simulink model "sampleModel2038"  (R2023a)
settings: Solver=VariableStepAuto  StartTime=0.0  StopTime=10.0  RelTol=1e-3
libraries: hdlsllib x8, simulink x2
settings Model: Creator=user1  LastModifiedBy=user1

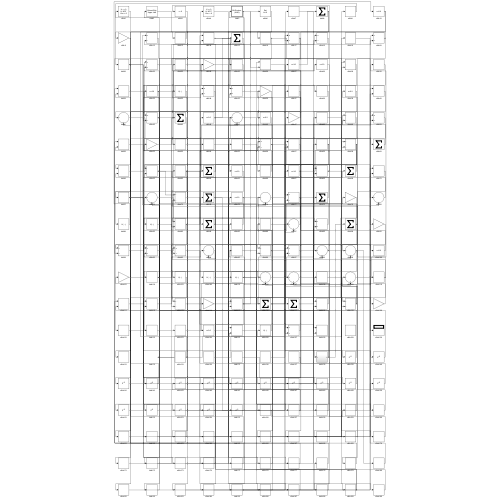
[thumbnail: Simulink's stored preview of the top-level diagram]
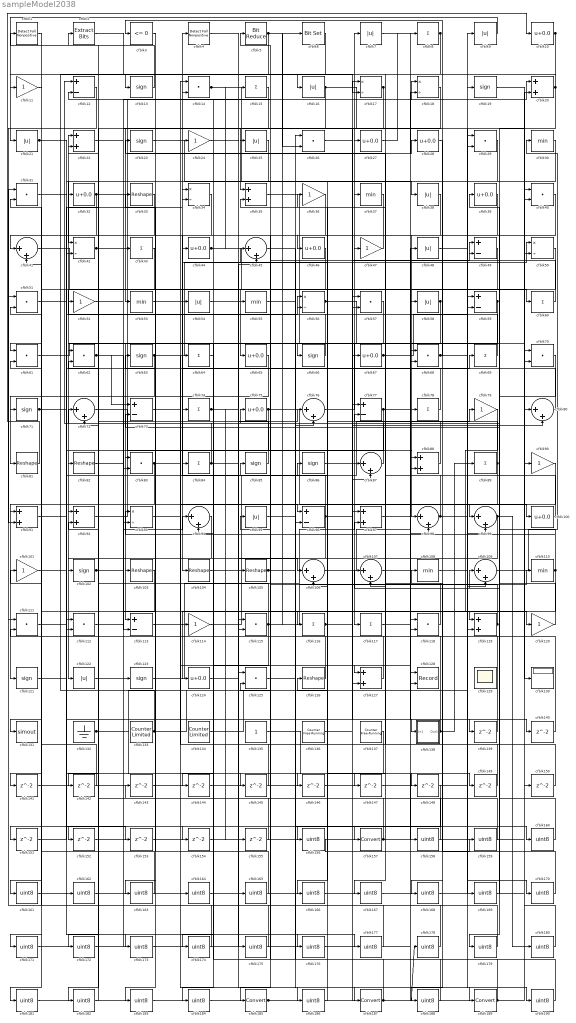
== system sampleModel2038 ==
  cfblk1 : hdlsllib/Logic and Bit Operations/Detect Fall Nonpositive  vinit=0  OutDataTypeStr=boolean
  cfblk{10,27..28,32,39,44,46,65,67,75,100,124} (12 alike) : Bias  Bias=0.0  SaturateOnIntegerOverflow=off
  cfblk{11,24,36,47,52,79,90,101,114,120} (10 alike) : Gain
  cfblk{13,19,23,63,66,71,85..86,102,121,123} (11 alike) : Signum
  cfblk{33,81..82,103..105,126} (7 alike) : Reshape
  cfblk{41,45,72,76,80,87,94,98..99,106..107,109} (12 alike) : Sum  Inputs=|++
  cfblk{30,37,53,55,108,110} (6 alike) : MinMax
  cfblk{14,26,29,31,40,51,57,61..62,68,70,83,111..112,115,118,125} (17 alike) : DotProduct  OutDataTypeStr=Inherit: Inherit via internal rule
  cfblk{12,49,59,73,77,96,113} (7 alike) : Sum  Inputs=+-
  cfblk{8,15,43,60,64,69,74,78,84,89,116..117} (12 alike) : Sum  Inputs=+
  cfblk{20,22,35,88,91..92,97,119,127} (9 alike) : Sum
  cfblk{7,9,16,21,25,38,48,54,58,95,122} (11 alike) : Abs  SaturateOnIntegerOverflow=off
  cfblk128 : Record  FileSettingsInternal="{\"entries\":[{\"content\":{\"excelSettings\":{\"content\":{},\"type\":\"Streamout.ExcelSettings\"}},\"type\":\"Streamout.FileSettingStorage\",\"uuid\":\"\"}],\"packageUris\":[\"http:\\/\\/schema.mathworks.com\\/mf0\\/streamout_blocks\\/R2020a\"],\"version\":\"1.0\"}"  Layout=[1 1]  SignalsInternal="{\"entries\":[{\"content\":{\"signals\":[{\"content\":{\"blockPath\":[],\"dimensions\":[1],\"domain\":\"\",\"lineColor\":\"#a2142f\",\"plots\":[1],\"port\":1,\"signalID\":6186,\"signalName\":\"XY Graph:1\"},\"type\":\"RecordBlkView.Signal\",\"uuid\":\"\"},{\"content\":{\"blockPath\":[],\"dimensions\":[1],\"domain\":\"\",\"lineColor\":\"#139fff\",\"plots\":[1],\"port\":2,\"signalID\":6189,\"signalName\":\"XY Graph:2\"},\"type\":\"RecordBlkView.Signal\",\"uuid\":\"\"}]},\"type\":\"RecordBlkView.InputSignals\",\"uuid\":\"\"}],\"packageUris\":[\"http:\\/\\/schema.mathworks.com\\/mf0\\/streamout_blocks\\/R2020a\"],\"version\":\"1.0\"}"  VisualizationBindings="{\"xyplotplugin\":{\"info\":[{\"series\":[{\"bindingParametersList\":[{\"parameter\":\"X-Axis\",\"signalID\":6186,\"signalName\":\"XY Graph:1\"},{\"parameter\":\"Y-Axis\",\"signalID\":6189,\"signalName\":\"XY Graph:2\"}],\"seriesID\":36534}],\"subplotID\":1}]}}"  CompatibilityTag=XY  st=-1
  cfblk129 : Scope
      settings: Floating=on
  cfblk130 : Display
  cfblk131 : ToWorkspace  VariableName=simout  SaveFormat=Timeseries  SampleTime=-1
  cfblk132 : Ground
  cfblk133 : hdlsllib/Sources/Counter Limited  uplimit=7  tsamp=-1
  cfblk134 : hdlsllib/Sources/Counter Limited  uplimit=7  tsamp=-1
  cfblk135 : Constant  SampleTime=-1
  cfblk136 : hdlsllib/Sources/Counter Free-Running  NumBits=16  tsamp=-1
  cfblk137 : hdlsllib/Sources/Counter Free-Running  NumBits=16  tsamp=-1
  cfblk138 : Subsystem
      settings: LibrarySourceBlock=|
      | hdlsllib/Ports &
      | Subsystems/Subsystem
  cfblk{139..155} (17 alike) : Delay  SampleTime=1
  cfblk{156,158..184,186,188,190} (31 alike) : DataTypeConversion  OutDataTypeStr=uint8  SaturateOnIntegerOverflow=off  RndMeth=Floor
  cfblk{157,185,187,189} (4 alike) : DataTypeConversion  SaturateOnIntegerOverflow=off  RndMeth=Floor
  cfblk{17..18,34,42,50,56,93} (7 alike) : Product  Inputs=*/  RndMeth=Zero  SaturateOnIntegerOverflow=on
  cfblk2 : simulink/Logic and Bit Operations/Extract Bits  bitsToExtract=Upper half  numBits=8  bitIdxRange=[0 7]  outScalingMode=Preserve fixed-point scaling
      settings: LibrarySourceBlock=|
      | hdlsllib/Logic and Bit
      | Operations/Extract Bits
  cfblk3 : hdlsllib/Logic and Bit Operations/Compare To Zero  relop=<=  OutDataTypeStr=boolean
  cfblk4 : hdlsllib/Logic and Bit Operations/Detect Fall Nonpositive  vinit=0  OutDataTypeStr=boolean
  cfblk5 : hdlsllib/Logic and Bit Operations/Bit Reduce  mode=AND
  cfblk6 : simulink/Logic and Bit Operations/Bit Set  iBit=0
      settings: LibrarySourceBlock=|
      | hdlsllib/Logic and Bit
      | Operations/Bit Set
  wires:
  cfblk27/1 -> cfblk8/1
  cfblk78/1 -> cfblk7/1
  cfblk85/1 -> cfblk22/1
  cfblk114/1 -> cfblk79/1
  cfblk98/1 -> cfblk27/1, cfblk109/2
  cfblk84/1 -> cfblk12/1, cfblk119/2
  cfblk133/1 -> cfblk13/1, cfblk45/2
  cfblk20/1 -> cfblk99/1, cfblk11/1
  cfblk68/1 -> cfblk3/1, cfblk170/1
  cfblk79/1 -> cfblk120/1
  cfblk89/1 -> cfblk121/1, cfblk44/1
  cfblk75/1 -> cfblk100/1, cfblk112/2
  cfblk96/1 -> cfblk4/1, cfblk128/2, cfblk144/1
  cfblk49/1 -> cfblk122/1
  cfblk9/1 -> cfblk21/1
  cfblk63/1 -> cfblk50/1, cfblk83/1, cfblk127/1, cfblk83/2
  cfblk87/1 -> cfblk75/1
  cfblk109/1 -> cfblk30/1
  cfblk92/1 -> cfblk28/1
  cfblk53/1 -> cfblk104/1
  cfblk18/1 -> cfblk82/1
  cfblk81/1 -> cfblk10/1
  cfblk80/1 -> cfblk34/1
  cfblk76/1 -> cfblk47/1
  cfblk15/1 -> cfblk35/1
  cfblk37/1 -> cfblk84/1
  cfblk69/1 -> cfblk22/2
  cfblk5/1 -> cfblk26/2, cfblk183/1
  cfblk50/1 -> cfblk65/1
  cfblk61/1 -> cfblk66/1
  cfblk42/1 -> cfblk18/1, cfblk142/1
  cfblk59/1 -> cfblk117/1, cfblk167/1, cfblk168/1
  cfblk35/1 -> cfblk130/1
  cfblk40/1 -> cfblk98/1
  cfblk58/1 -> cfblk113/1, cfblk114/1
  cfblk115/1 -> cfblk110/1, cfblk6/1, cfblk72/1, cfblk184/1
  cfblk13/1 -> cfblk1/1
  cfblk65/1 -> cfblk81/1
  cfblk23/1 -> cfblk77/1
  cfblk119/1 -> cfblk5/1, cfblk107/1
  cfblk21/1 -> cfblk145/1, cfblk146/1
  cfblk17/1 -> cfblk53/1, cfblk127/2
  cfblk19/1 -> cfblk80/1
  cfblk10/1 -> cfblk91/1, cfblk115/2
  cfblk3/1 -> cfblk103/1
  cfblk47/1 -> cfblk41/1
  cfblk46/1 -> cfblk102/1
  cfblk88/1 -> cfblk37/1
  cfblk134/1 -> cfblk59/1
  cfblk102/1 -> cfblk94/1, cfblk62/2
  cfblk120/1 -> cfblk74/1
  cfblk14/1 -> cfblk38/1, cfblk50/2
  cfblk99/1 -> cfblk152/1, cfblk180/1
  cfblk118/1 -> cfblk23/1
  cfblk1/1 -> cfblk131/1
  cfblk22/1 -> cfblk25/1
  cfblk138/1(Out1) -> cfblk63/1, cfblk72/2, cfblk89/1
  cfblk116/1 -> cfblk49/1, cfblk80/2
  cfblk7/1 -> cfblk128/1
  cfblk32/1 -> cfblk18/2, cfblk61/1
  cfblk83/1 -> cfblk56/1, cfblk93/2
  cfblk104/1 -> cfblk76/1
  cfblk60/1 -> cfblk12/2
  cfblk34/1 -> cfblk92/1
  cfblk67/1 -> cfblk19/1, cfblk107/2
  cfblk132/1 -> cfblk97/1, cfblk175/1
  cfblk100/1 -> cfblk35/2
  cfblk30/1 -> cfblk42/1
  cfblk112/1 -> cfblk20/1
  cfblk77/1 -> cfblk48/1, cfblk94/2
  cfblk71/1 -> cfblk138/1(In1), cfblk34/2, cfblk153/1
  cfblk127/1 -> cfblk92/2
  cfblk123/1 -> cfblk97/2
  cfblk136/1 -> cfblk67/1
  cfblk122/1 -> cfblk123/1
  cfblk73/1 -> cfblk96/1
  cfblk91/1 -> cfblk69/1
  cfblk64/1 -> cfblk14/2
  cfblk62/1 -> cfblk119/1, cfblk73/1
  cfblk11/1 -> cfblk71/1
  cfblk16/1 -> cfblk59/2, cfblk62/1
  cfblk24/1 -> cfblk187/1
  cfblk107/1 -> cfblk68/1
  cfblk126/1 -> cfblk32/1
  cfblk44/1 -> cfblk90/1, cfblk15/1
  cfblk12/1 -> cfblk91/2
  cfblk26/1 -> cfblk60/1
  cfblk74/1 -> cfblk106/1, cfblk155/1
  cfblk41/1 -> cfblk87/2
  cfblk95/1 -> cfblk189/1
  cfblk105/1 -> cfblk148/1, cfblk149/1
  cfblk38/1 -> cfblk46/1
  cfblk51/1 -> cfblk56/2
  cfblk36/1 -> cfblk185/1
  cfblk8/1 -> cfblk16/1, cfblk147/1
  cfblk82/1 -> cfblk113/2
  cfblk72/1 -> cfblk88/1
  cfblk106/1 -> cfblk49/2
  cfblk56/1 -> cfblk116/1, cfblk118/1
  cfblk113/1 -> cfblk124/1
  cfblk52/1 -> cfblk54/1
  cfblk54/1 -> cfblk96/2
  cfblk125/1 -> cfblk157/1
  cfblk110/1 -> cfblk73/2, cfblk93/1, cfblk174/1
  cfblk66/1 -> cfblk45/1
  cfblk121/1 -> cfblk85/1
  cfblk2/1 -> cfblk17/2
  cfblk25/1 -> cfblk42/2
  cfblk117/1 -> cfblk88/2
  cfblk45/1 -> cfblk68/2
  cfblk97/1 -> cfblk139/1
  cfblk139/1 -> cfblk41/2
  cfblk86/1 -> cfblk140/1
  cfblk140/1 -> cfblk51/2
  cfblk39/1 -> cfblk141/1
  cfblk141/1 -> cfblk76/2
  cfblk142/1 -> cfblk61/2
  cfblk144/1 -> cfblk118/2
  cfblk145/1 -> cfblk14/1
  cfblk146/1 -> cfblk98/2
  cfblk147/1 -> cfblk99/2
  cfblk149/1 -> cfblk77/2
  cfblk150/1 -> cfblk115/1
  cfblk6/1 -> cfblk151/1
  cfblk151/1 -> cfblk112/1
  cfblk152/1 -> cfblk20/2
  cfblk153/1 -> cfblk87/1
  cfblk90/1 -> cfblk154/1
  cfblk154/1 -> cfblk17/1
  cfblk155/1 -> cfblk33/1
  cfblk137/1 -> cfblk156/1
  cfblk157/1 -> cfblk2/1, cfblk106/2
  cfblk135/1 -> cfblk158/1
  cfblk158/1 -> cfblk125/1
  cfblk156/1 -> cfblk159/1
  cfblk159/1 -> cfblk125/2
  cfblk55/1 -> cfblk160/1
  cfblk160/1 -> cfblk39/1
  cfblk103/1 -> cfblk161/1
  cfblk161/1 -> cfblk55/1
  cfblk101/1 -> cfblk162/1
  cfblk162/1 -> cfblk40/2
  cfblk94/1 -> cfblk163/1
  cfblk163/1 -> cfblk101/1
  cfblk143/1 -> cfblk164/1
  cfblk164/1 -> cfblk40/1
  cfblk4/1 -> cfblk165/1
  cfblk165/1 -> cfblk143/1
  cfblk29/1 -> cfblk166/1
  cfblk166/1 -> cfblk9/1
  cfblk167/1 -> cfblk29/1
  cfblk168/1 -> cfblk29/2
  cfblk108/1 -> cfblk169/1
  cfblk169/1 -> cfblk109/1
  cfblk170/1 -> cfblk108/1
  cfblk43/1 -> cfblk171/1
  cfblk171/1 -> cfblk58/1
  cfblk33/1 -> cfblk172/1
  cfblk172/1 -> cfblk43/1
  cfblk111/1 -> cfblk173/1
  cfblk173/1 -> cfblk105/1
  cfblk174/1 -> cfblk111/1
  cfblk175/1 -> cfblk111/2
  cfblk31/1 -> cfblk176/1
  cfblk176/1 -> cfblk86/1
  cfblk124/1 -> cfblk177/1
  cfblk177/1 -> cfblk31/1
  cfblk178/1 -> cfblk31/2
  cfblk70/1 -> cfblk179/1
  cfblk179/1 -> cfblk51/1
  cfblk180/1 -> cfblk70/1
  cfblk148/1 -> cfblk181/1
  cfblk181/1 -> cfblk70/2
  cfblk57/1 -> cfblk182/1
  cfblk182/1 -> cfblk52/1
  cfblk183/1 -> cfblk57/1
  cfblk184/1 -> cfblk57/2
  cfblk185/1 -> cfblk150/1, cfblk78/1
  cfblk93/1 -> cfblk186/1
  cfblk186/1 -> cfblk36/1
  cfblk187/1 -> cfblk178/1, cfblk126/1
  cfblk28/1 -> cfblk188/1
  cfblk188/1 -> cfblk24/1
  cfblk189/1 -> cfblk26/1, cfblk64/1
  cfblk48/1 -> cfblk190/1
  cfblk190/1 -> cfblk95/1

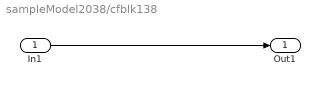
== system sampleModel2038/cfblk138 ==
  In1 : Inport
  Out1 : Outport
  wires:
  In1/1 -> Out1/1
